simulink model "pitch_3dof"  (R2022b)
settings: Solver=VariableStepAuto  StartTime=0.0  StopTime=50.0  RelTol=1e-3
libraries: simulink_extras x1
settings Model: Creator=Tejal Mahajan  LastModifiedBy=Tejal Mahajan

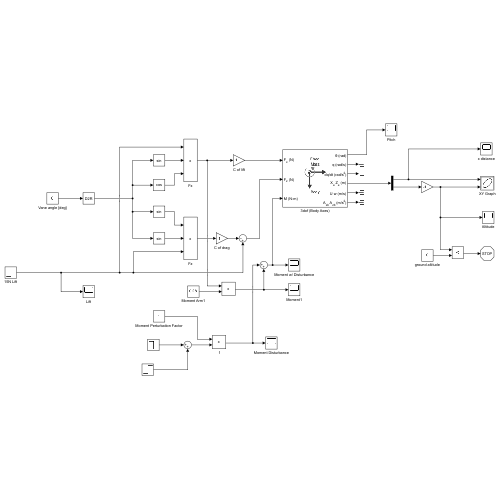
[thumbnail: Simulink's stored preview of the top-level diagram]
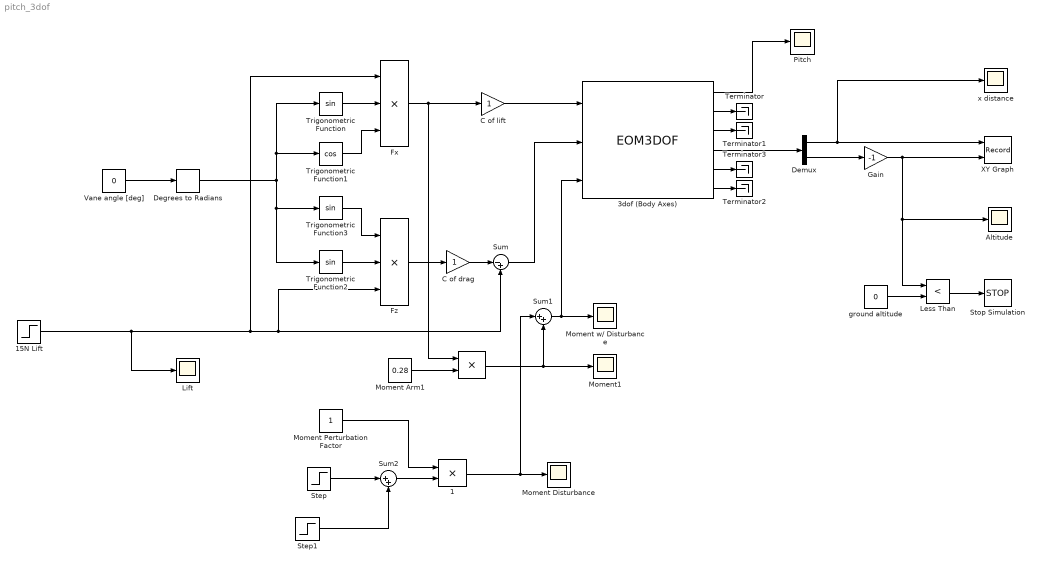
== system pitch_3dof ==
  " " : Product
  " 1" : Product
  15N Lift : Step  Time=10  Before=-6  After=-5  SampleTime=0
  3dof (Body Axes) : EOM3DOF  v_ini=0  mass=0.543  Iyy=0.048  vel_statename={'u', 'w'}  pos_statename={'Xe', 'Ze'}  q_statename='omega'  theta_statename='theta'
  Altitude : Scope
  C of drag : Gain
  C of lift : Gain
  Degrees to Radians : simulink_extras/Transformations/Degrees to Radians
  Demux : Demux  Outputs=2
  Fx : Product  Inputs=3
  Fz : Product  Inputs=3
  Gain : Gain  Gain=-1
  Less Than : RelationalOperator  Operator=<  OutDataTypeStr=boolean  RndMeth=Simplest  InputSameDT=off
  Lift : Scope
  Moment Arm1 : Constant  Value=0.28
  Moment Disturbance : Scope
  Moment Perturbation Factor : Constant
  Moment w/ Disturbance : Scope
  Moment1 : Scope
  Pitch : Scope
  Step : Step  Time=3  After=-1e-7  SampleTime=0
  Step1 : Step  Time=2  After=1e-7  SampleTime=0
  Stop Simulation : Stop
  Sum : Sum  Inputs=|-+
  Sum1 : Sum  Inputs=|++
  Sum2 : Sum  Inputs=|++
  Terminator{,1..3} (4 alike) : Terminator
  Trigonometric Function : Trigonometry
  Trigonometric Function1 : Trigonometry  Operator=cos
  Trigonometric Function2 : Trigonometry
  Trigonometric Function3 : Trigonometry
  Vane angle [deg] : Constant  Value=0
  XY Graph : Record  FileSettingsInternal="{\"entries\":[{\"content\":{\"excelSettings\":{\"content\":{},\"type\":\"Streamout.ExcelSettings\"}},\"type\":\"Streamout.FileSettingStorage\",\"uuid\":\"83fdc34a-714a-41c0-ba65-9d684819995a\"}],\"packageUris\":[\"http://schema.mathworks.com/mf0/streamout_blocks/R2020a\"],\"version\":\"1.0\"}"  Layout=[1 1]  SignalsInternal="{\"entries\":[{\"content\":{\"signals\":[{\"content\":{\"blockPath\":[\"pitch_3dof/XY Graph\"],\"channel\":[],\"dimensions\":[1],\"domain\":\"pitch_3dof/XY Graph\",\"lineColor\":\"#edb120\",\"plots\":[],\"port\":1,\"sid\":[\"\"],\"signalID\":944,\"signalName\":\"Demux:1\"},\"type\":\"RecordBlkView.Signal\",\"uuid\":\"1d2c49b1-9649-4386-851a-852d3304b6fc\"},{\"content\":{\"blockPath\":[\"pitch_3dof/XY Graph\"],\"channel\":[],\"dimensions\":[1],\"domain\":\"pitch_3dof/XY Graph\",\"lineColor\":\"#7e2f8e\",\"plots\":[],\"port\":2,\"sid\":[\"\"],\"signalID\":948,\"signalName\":\"Gain\"},\"type\":\"RecordBlkView.Signal\",\"uuid\":\"1b564bb3-4e7f-460f-81a9-e8c78b445eb1\"}]},\"type\":\"RecordBlkView.InputSignals\",\"uuid\":\"b63abfb6-e3ba-4317-8f35-f35550fcf14c\"}],\"packageUris\":[\"http://schema.mathworks.com/mf0/streamout_blocks/R2020a\"],\"version\":\"1.0\"}"  VisualizationBindings="{\"xyplotplugin\":{\"info\":[{\"series\":[],\"subplotID\":1}]}}"  CompatibilityTag=XY
  ground altitude : Constant  Value=0
  x distance : Scope
  wires:
  Vane angle [deg]/1 -> Degrees to Radians/1
  Trigonometric Function/1 -> Fx/2
  Trigonometric Function1/1 -> Fx/3
  Trigonometric Function2/1 -> Fz/2
  Trigonometric Function3/1 -> Fz/1
  Degrees to Radians/1 -> Trigonometric Function2/1, Trigonometric Function3/1, Trigonometric Function1/1, Trigonometric Function/1
  15N Lift/1 -> Lift/1, Fx/1, Fz/3, Sum/2
  Fx/1 -> C of lift/1, " "/1
  Sum/1 -> 3dof (Body Axes)/2
  Moment Arm1/1 -> " "/2
  " "/1 -> Sum1/2, Moment1/1
  Sum1/1 -> Moment w/ Disturbance/1, 3dof (Body Axes)/3
  Step/1 -> Sum2/1
  Step1/1 -> Sum2/2
  Sum2/1 -> " 1"/2
  Moment Perturbation Factor/1 -> " 1"/1
  " 1"/1 -> Moment Disturbance/1, Sum1/1
  3dof (Body Axes)/1 -> Pitch/1
  3dof (Body Axes)/2 -> Terminator/1
  3dof (Body Axes)/5 -> Terminator3/1
  3dof (Body Axes)/6 -> Terminator2/1
  3dof (Body Axes)/3 -> Terminator1/1
  3dof (Body Axes)/4 -> Demux/1
  Demux/2 -> Gain/1
  Gain/1 -> Altitude/1, Less Than/1, XY Graph/2
  Demux/1 -> x distance/1, XY Graph/1
  ground altitude/1 -> Less Than/2
  Less Than/1 -> Stop Simulation/1
  C of lift/1 -> 3dof (Body Axes)/1
  C of drag/1 -> Sum/1
  Fz/1 -> C of drag/1
